simulink model "Question6"  (R2017b)
settings: Solver=VariableStepAuto  StartTime=0.0  StopTime=10.0  RelTol=1e-3
settings Model: Creator=Ray  LastModifiedBy=Ray

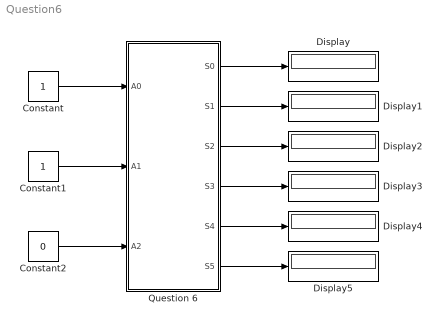
== system Question6 ==
  Constant : Constant  OutDataTypeStr=boolean  SampleTime=1
  Constant1 : Constant  OutDataTypeStr=boolean  SampleTime=1
  Constant2 : Constant  Value=0  OutDataTypeStr=boolean  SampleTime=1
  Display{,1..5} (6 alike) : Display
  Question 6 : Subsystem
  wires:
  Question 6/1(S0) -> Display/1
  Question 6/2(S1) -> Display1/1
  Question 6/3(S2) -> Display2/1
  Question 6/4(S3) -> Display3/1
  Question 6/5(S4) -> Display4/1
  Question 6/6(S5) -> Display5/1
  Constant/1 -> Question 6/1(A0)
  Constant1/1 -> Question 6/2(A1)
  Constant2/1 -> Question 6/3(A2)

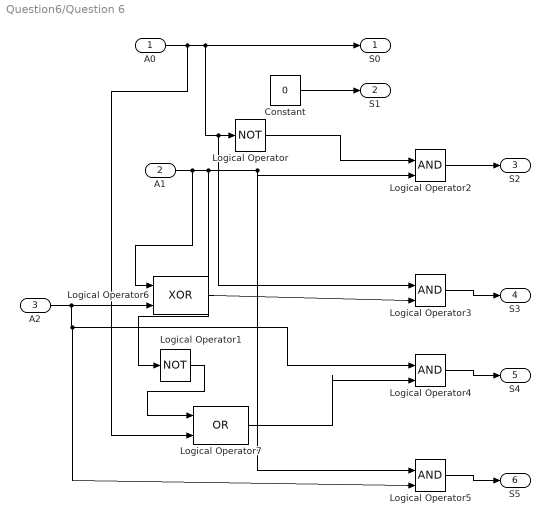
== system Question6/Question 6 ==
  A0 : Inport  OutDataTypeStr=boolean  SampleTime=1
  A1 : Inport  Port=2  OutDataTypeStr=boolean  SampleTime=1
  A2 : Inport  Port=3  OutDataTypeStr=boolean  SampleTime=1
  Constant : Constant  Value=0  OutDataTypeStr=boolean  SampleTime=1
  Logical Operator : Logic  Operator=NOT  IconShape=distinctive  AllPortsSameDT=off  OutDataTypeStr=boolean
  Logical Operator1 : Logic  Operator=NOT  IconShape=distinctive  AllPortsSameDT=off  OutDataTypeStr=boolean
  Logical Operator{2..5} (4 alike) : Logic  IconShape=distinctive  AllPortsSameDT=off  OutDataTypeStr=boolean
  Logical Operator6 : Logic  Operator=XOR  IconShape=distinctive  AllPortsSameDT=off  OutDataTypeStr=boolean
  Logical Operator7 : Logic  Operator=OR  IconShape=distinctive  AllPortsSameDT=off  OutDataTypeStr=boolean
  S0 : Outport  OutDataTypeStr=boolean  SampleTime=1
  S1 : Outport  Port=2  OutDataTypeStr=boolean  SampleTime=1
  S2 : Outport  Port=3  OutDataTypeStr=boolean  SampleTime=1
  S3 : Outport  Port=4  OutDataTypeStr=boolean  SampleTime=1
  S4 : Outport  Port=5  OutDataTypeStr=boolean  SampleTime=1
  S5 : Outport  Port=6  OutDataTypeStr=boolean  SampleTime=1
  wires:
  Logical Operator2/1 -> S2/1
  Logical Operator5/1 -> S5/1
  Logical Operator7/1 -> Logical Operator4/2
  A0/1 -> S0/1, Logical Operator3/1, Logical Operator/1, Logical Operator7/2
  A1/1 -> Logical Operator6/1, Logical Operator5/1, Logical Operator2/2, Logical Operator1/1
  A2/1 -> Logical Operator5/2, Logical Operator4/1, Logical Operator6/2
  Logical Operator1/1 -> Logical Operator7/1
  Logical Operator3/1 -> S3/1
  Logical Operator6/1 -> Logical Operator3/2
  Logical Operator/1 -> Logical Operator2/1
  Logical Operator4/1 -> S4/1
  Constant/1 -> S1/1
